simulink model "OMSv1_2x"  (Simulink 6.5)
settings: Solver=ode4  SolverMode=SingleTasking  StartTime=0.0  StopTime=5  FixedStep=0.001  MaxStep=0.001  RelTol=1e-3  AbsTol=1e-3
undefined symbols (not defined in the file): alexlaw, bs_onoff, bs_scale, bsfsacrit, bsfsvcrit, cnsgain, fs_onoff, fs_scale, fsdelaycalc, ltdrk, phasicgain, pmcgain, pmctau2, pmctau3, saccsw, spgain, tonicgain, tvrD, tvrN
libraries: simulink_extras x37
(part 4 of 5)

== system OMSv1_2x/OMS v1.2  07/21/05/IM CN-LMLN/Saccade Enable/Ret FB sample/event timer2 ==
  note: Resettable
      | Event Timer
  note: (Init input: 0)
  note: (FF init state: Q=0)
  note: (Init input: 0)
  note: In 2) Subsequent events DO NOT reset the counter; it only resets when it
      | reaches zero
  note: 2) A new event (leading or trailing edge) is detected. -- Only case 1)
  note: 1) The count reaches its limit (set in "timer value") -- Both case 1) and 2)
  note: In 1), A leading or trailing edge will reset the counter so that it
      | counts down from the end trailing edge) of that event.
  note: It has TWO modes: 1) Event resettable and 2) Event Non-resettable
  note: The real trick here is understanding how to reload the countdown.
      | It resets if either of two conditions is met:
  note: The "OR" gate allows either of these conditions to reset the circuit.  The delay before the
      | "S" input of the flip-flop prevents both "S" and "R" from being set simultaneously, because
      | this would put the flip-flop in an undefined state.
  note: Therefore, an event first RESETS and then SETS the flip-flop.
  note: This block is an RESETTABLE EVENT TIMER.  It outputs a spike of unit height xx milliseconds
      | (set by "timer value") after it detects an event ( i.e a TRAILING edge which represents the end of a
      |  saccadic pulse)
  RetFB EnCntrl : Inport
  _timer value (port) : Inport  Port=2
  1 msec : TransportDelay  DelayTime=.001
  Clock : Clock
      settings: Decimation=10
  Latch1 : simulink_extras/Flip Flops/S-R Flip-Flop  SystemSampleTime=-1  initial_condition=0
  Logical Operator : Logic  Operator=OR  Inputs=3
  Logical Operator1 : Logic
  Logical Operator2 : Logic
  Relational Operator : RelationalOperator  InputSameDT=on
  SampHold?1 : Subsystem
      mask Display: disp('S&H\n(S=L)\n(H=H)')
  Sum : Sum  Inputs=+-  SaturateOnIntegerOverflow=on  InputSameDT=on
  Terminator : Terminator
  event resettable? : Constant  Orientation=up
  leading edge detect : Subsystem
      mask Display: disp('Leading\nEdge Det')
  loop breaker : Memory  Orientation=left
  trailing edge detect : Subsystem
      mask Display: disp('Trailing\nEdge Det')
  outFF : Outport  InitialOutput=0
  wires:
  RetFB EnCntrl/1 -> trailing edge detect/1(in_1), leading edge detect/1(in_1)
  event resettable?/1 -> Logical Operator1/2, Logical Operator2/2
  leading edge detect/1(out_1) -> Logical Operator2/1
  Logical Operator2/1 -> Logical Operator/2
  trailing edge detect/1(out_1) -> 1 msec/1, Logical Operator1/1
  Logical Operator1/1 -> Logical Operator/1
  loop breaker/1 -> Logical Operator/3
  Latch1/1 -> SampHold?1/2(S/H?)
  Sum/1 -> Relational Operator/1
  Clock/1 -> SampHold?1/1(Input), Sum/1
  Relational Operator/1 -> outFF/1, loop breaker/1
  SampHold?1/1(output) -> Sum/2
  Logical Operator/1 -> Latch1/2
  1 msec/1 -> Latch1/1
  _timer value (port)/1 -> Relational Operator/2
  Latch1/2 -> Terminator/1

== system OMSv1_2x/OMS v1.2  07/21/05/IM CN-LMLN/Saccade Enable/Ret FB sample/event timer3 ==
  note: This block is an RESETTABLE EVENT TIMER.  It outputs a spike of unit height xx milliseconds
      | (set by "timer value") after it detects an event ( i.e a TRAILING edge which represents the end of a
      |  saccadic pulse)
  note: Therefore, an event first RESETS and then SETS the flip-flop.
  note: The "OR" gate allows either of these conditions to reset the circuit.  The delay before the
      | "S" input of the flip-flop prevents both "S" and "R" from being set simultaneously, because
      | this would put the flip-flop in an undefined state.
  note: The real trick here is understanding how to reload the countdown.
      | It resets if either of two conditions is met:
  note: It has TWO modes: 1) Event resettable and 2) Event Non-resettable
  note: In 1), A leading or trailing edge will reset the counter so that it
      | counts down from the end trailing edge) of that event.
  note: 1) The count reaches its limit (set in "timer value") -- Both case 1) and 2)
  note: 2) A new event (leading or trailing edge) is detected. -- Only case 1)
  note: In 2) Subsequent events DO NOT reset the counter; it only resets when it
      | reaches zero
  note: (Init input: 0)
  note: (FF init state: Q=0)
  note: (Init input: 0)
  note: Resettable
      | Event Timer
  RetFB EnCntrl : Inport
  _timer value (port) : Inport  Port=2
  1 msec : TransportDelay  DelayTime=.001
  Clock : Clock
      settings: Decimation=10
  Latch1 : simulink_extras/Flip Flops/S-R Flip-Flop  SystemSampleTime=-1  initial_condition=0
  Logical Operator : Logic  Operator=OR  Inputs=3
  Logical Operator1 : Logic
  Logical Operator2 : Logic
  Relational Operator : RelationalOperator  InputSameDT=on
  SampHold?1 : Subsystem
      mask Display: disp('S&H\n(S=L)\n(H=H)')
  Sum : Sum  Inputs=+-  SaturateOnIntegerOverflow=on  InputSameDT=on
  Terminator : Terminator
  event resettable? : Constant  Orientation=up
  leading edge detect : Subsystem
      mask Display: disp('Leading\nEdge Det')
  loop breaker : Memory  Orientation=left
  trailing edge detect : Subsystem
      mask Display: disp('Trailing\nEdge Det')
  outFF : Outport  InitialOutput=0
  wires:
  _timer value (port)/1 -> Relational Operator/2
  1 msec/1 -> Latch1/1
  Logical Operator/1 -> Latch1/2
  SampHold?1/1(output) -> Sum/2
  Clock/1 -> SampHold?1/1(Input), Sum/1
  Sum/1 -> Relational Operator/1
  Relational Operator/1 -> loop breaker/1, outFF/1
  Latch1/1 -> SampHold?1/2(S/H?)
  loop breaker/1 -> Logical Operator/3
  Logical Operator1/1 -> Logical Operator/1
  trailing edge detect/1(out_1) -> 1 msec/1, Logical Operator1/1
  Logical Operator2/1 -> Logical Operator/2
  leading edge detect/1(out_1) -> Logical Operator2/1
  event resettable?/1 -> Logical Operator1/2, Logical Operator2/2
  RetFB EnCntrl/1 -> trailing edge detect/1(in_1), leading edge detect/1(in_1)
  Latch1/2 -> Terminator/1

== system OMSv1_2x/OMS v1.2  07/21/05/IM CN-LMLN/Saccade Enable/Ret FB sample/leading edge detect2 ==
  note: It is also possible to remove the SIGNUM function
      | and the '==', and replace them with a simple
      | switch with a threshold of (say) 150 or so.
  note: leading edge detection
  in_1 : Inport
  Abs : Abs  SaturateOnIntegerOverflow=on
  Derivative : Derivative
  Relational Operator : RelationalOperator  Operator===  InputSameDT=on
  Sign : Signum
  Threshold 1 : Constant
  out_1 : Outport  InitialOutput=0
  wires:
  Abs/1 -> Derivative/1
  Derivative/1 -> Sign/1
  Sign/1 -> Relational Operator/1
  Threshold 1/1 -> Relational Operator/2
  Relational Operator/1 -> out_1/1
  in_1/1 -> Abs/1

== system OMSv1_2x/OMS v1.2  07/21/05/IM CN-LMLN/Saccade Enable/Ret FB sample/leading edge detect3 ==
  note: leading edge detection
  note: It is also possible to remove the SIGNUM function
      | and the '==', and replace them with a simple
      | switch with a threshold of (say) 150 or so.
  in_1 : Inport
  Abs : Abs  SaturateOnIntegerOverflow=on
  Derivative : Derivative
  Relational Operator : RelationalOperator  Operator===  InputSameDT=on
  Sign : Signum
  Threshold 1 : Constant
  out_1 : Outport  InitialOutput=0
  wires:
  in_1/1 -> Abs/1
  Relational Operator/1 -> out_1/1
  Threshold 1/1 -> Relational Operator/2
  Sign/1 -> Relational Operator/1
  Derivative/1 -> Sign/1
  Abs/1 -> Derivative/1

== system OMSv1_2x/OMS v1.2  07/21/05/IM CN-LMLN/Saccade Enable/Ret FB sample/leading edge detect4 ==
  note: It is also possible to remove the SIGNUM function
      | and the '==', and replace them with a simple
      | switch with a threshold of (say) 150 or so.
  note: leading edge detection
  in_1 : Inport
  Abs : Abs  SaturateOnIntegerOverflow=on
  Derivative : Derivative
  Relational Operator : RelationalOperator  Operator===  InputSameDT=on
  Sign : Signum
  Threshold 1 : Constant
  out_1 : Outport  InitialOutput=0
  wires:
  Abs/1 -> Derivative/1
  Derivative/1 -> Sign/1
  Sign/1 -> Relational Operator/1
  Threshold 1/1 -> Relational Operator/2
  Relational Operator/1 -> out_1/1
  in_1/1 -> Abs/1

== system OMSv1_2x/OMS v1.2  07/21/05/IM CN-LMLN/Saccade Enable/prolong/SampHold?2 ==
  note: When "S/H?" is LOW, then "Input" is switched directly to the
      | output ("sample").  When "S/H?" is HIGH, the current output is
      | maintained ("hold").
  Input : Inport
  S/H? : Inport  Port=2
  Memory : Memory  Orientation=left
  Sign : Signum
  Switch2 : Switch  Threshold=0.5  SaturateOnIntegerOverflow=on  InputSameDT=on
  output : Outport  InitialOutput=0
  wires:
  Memory/1 -> Switch2/1
  Switch2/1 -> output/1, Memory/1
  Input/1 -> Switch2/3
  Sign/1 -> Switch2/2
  S/H?/1 -> Sign/1

== system OMSv1_2x/OMS v1.2  07/21/05/IM CN-LMLN/Saccade Enable/prolong/leading edge detect ==
  note: leading edge detection
  in_1 : Inport
  Abs : Abs  SaturateOnIntegerOverflow=on
  Derivative : Derivative
  Relational Operator : RelationalOperator  Operator===  InputSameDT=on
  Sign : Signum
  Threshold 1 : Constant
  out_1 : Outport  InitialOutput=0
  wires:
  Abs/1 -> Derivative/1
  Derivative/1 -> Sign/1
  Sign/1 -> Relational Operator/1
  Threshold 1/1 -> Relational Operator/2
  Relational Operator/1 -> out_1/1
  in_1/1 -> Abs/1

== system OMSv1_2x/OMS v1.2  07/21/05/IM CN-LMLN/Saccade Enable/prolong/trailing edge detect ==
  note: trailing edge detection
  note: It is also possible to remove the SIGNUM function
      | and the '==', and replace them with a simple
      | switch with a threshold of (say) 150 or so.
  in_1 : Inport
  Abs : Abs  SaturateOnIntegerOverflow=on
  Derivative : Derivative
  Relational Operator : RelationalOperator  Operator===  InputSameDT=on
  Sign : Signum
  Threshold 1 : Constant  Value=-1
  out_1 : Outport  InitialOutput=0
  wires:
  in_1/1 -> Abs/1
  Relational Operator/1 -> out_1/1
  Threshold 1/1 -> Relational Operator/2
  Sign/1 -> Relational Operator/1
  Derivative/1 -> Sign/1
  Abs/1 -> Derivative/1

== system OMSv1_2x/OMS v1.2  07/21/05/IM CN-LMLN/Saccade Motor Commmand/TCHNG Override/event timer2 ==
  note: In 2) Subsequent events DO NOT reset the counter; it only resets when it
      | reaches zero
  note: 2) A new event (leading or trailing edge) is detected. -- Only case 1)
  note: 1) The count reaches its limit (set in "timer value") -- Both case 1) and 2)
  note: In 1), Any event (leading or trailing edge) will reset the counter so that it
      | counts down from the end trailing edge) of that event.
  note: It has TWO modes: 1) Event resettable and 2) Event Non-resettable
  note: The real trick here is understanding how to reload the countdown.
      | It resets if either of two conditions is met:
  note: The "OR" gate allows either of these conditions to reset the circuit.  The delay before the
      | "S" input of the flip-flop prevents both "S" and "R" from being set simultaneously, because
      | this would put the flip-flop in an undefined state.
  note: Therefore, an event first RESETS and then SETS the flip-flop.
  note: (Init input: 0)
  note: (FF init state: Q=0)
  note: (Init input: 0)
  note: This block is an RESETTABLE EVENT TIMER.  It outputs a spike of unit height xx milliseconds
      | (set by "timer value") after it detects an event ( i.e a TRAILING edge which represents the end of a
      |  saccadic pulse)
  note: Resettable
      | Event Timer
  _PG : Inport
  _timer value (port) : Inport  Port=2
  1 msec : TransportDelay  DelayTime=.001
  Clock : Clock
      settings: Decimation=10
  Latch1 : simulink_extras/Flip Flops/S-R Flip-Flop  SystemSampleTime=-1  initial_condition=0
  Logical Operator : Logic  Operator=OR  Inputs=3
  Logical Operator1 : Logic
  Logical Operator2 : Logic
  Relational Operator : RelationalOperator  InputSameDT=on
  SampHold?1 : Subsystem
      mask Display: disp('S&H\n(S=L)\n(H=H)')
  Sum : Sum  Inputs=+-  SaturateOnIntegerOverflow=on  InputSameDT=on
  Terminator : Terminator
  event resettable? : Constant  Orientation=up  Value=0
  leading edge detect : Subsystem
      mask Display: disp('Leading\nEdge Det')
  loop breaker : Memory  Orientation=left
  trailing edge detect : Subsystem
      mask Display: disp('Trailing\nEdge Det')
  out_1 : Outport  InitialOutput=0
  wires:
  event resettable?/1 -> Logical Operator2/2, Logical Operator1/2
  leading edge detect/1(out_1) -> Logical Operator2/1
  Logical Operator2/1 -> Logical Operator/2
  trailing edge detect/1(out_1) -> Logical Operator1/1, 1 msec/1
  Logical Operator1/1 -> Logical Operator/1
  loop breaker/1 -> Logical Operator/3
  _PG/1 -> leading edge detect/1(in_1), trailing edge detect/1(in_1)
  Latch1/1 -> SampHold?1/2(S/H?)
  Relational Operator/1 -> out_1/1, loop breaker/1
  Sum/1 -> Relational Operator/1
  Clock/1 -> Sum/1, SampHold?1/1(Input)
  SampHold?1/1(output) -> Sum/2
  Logical Operator/1 -> Latch1/2
  1 msec/1 -> Latch1/1
  _timer value (port)/1 -> Relational Operator/2
  Latch1/2 -> Terminator/1

== system OMSv1_2x/OMS v1.2  07/21/05/IM CN-LMLN/Saccade Motor Commmand/TCHNG Override/leading edge detect ==
  note: leading edge detection
  in_1 : Inport
  Abs : Abs  SaturateOnIntegerOverflow=on
  Derivative : Derivative
  Relational Operator : RelationalOperator  Operator===  InputSameDT=on
  Sign : Signum
  Threshold 1 : Constant
  out_1 : Outport  InitialOutput=0
  wires:
  in_1/1 -> Abs/1
  Relational Operator/1 -> out_1/1
  Threshold 1/1 -> Relational Operator/2
  Sign/1 -> Relational Operator/1
  Derivative/1 -> Sign/1
  Abs/1 -> Derivative/1

== system OMSv1_2x/OMS v1.2  07/21/05/IM CN-LMLN/Sampled Target Reconstruction/prolong/SampHold?2 ==
  note: When "S/H?" is LOW, then "Input" is switched directly to the
      | output ("sample").  When "S/H?" is HIGH, the current output is
      | maintained ("hold").
  Input : Inport
  S/H? : Inport  Port=2
  Memory : Memory  Orientation=left
  Sign : Signum
  Switch2 : Switch  Threshold=0.5  SaturateOnIntegerOverflow=on  InputSameDT=on
  output : Outport  InitialOutput=0
  wires:
  S/H?/1 -> Sign/1
  Sign/1 -> Switch2/2
  Input/1 -> Switch2/3
  Switch2/1 -> Memory/1, output/1
  Memory/1 -> Switch2/1

== system OMSv1_2x/OMS v1.2  07/21/05/IM CN-LMLN/Sampled Target Reconstruction/prolong/leading edge detect ==
  note: leading edge detection
  in_1 : Inport
  Abs : Abs  SaturateOnIntegerOverflow=on
  Derivative : Derivative
  Relational Operator : RelationalOperator  Operator===  InputSameDT=on
  Sign : Signum
  Threshold 1 : Constant
  out_1 : Outport  InitialOutput=0
  wires:
  in_1/1 -> Abs/1
  Relational Operator/1 -> out_1/1
  Threshold 1/1 -> Relational Operator/2
  Sign/1 -> Relational Operator/1
  Derivative/1 -> Sign/1
  Abs/1 -> Derivative/1

== system OMSv1_2x/OMS v1.2  07/21/05/IM CN-LMLN/Sampled Target Reconstruction/prolong/trailing edge detect ==
  note: It is also possible to remove the SIGNUM function
      | and the '==', and replace them with a simple
      | switch with a threshold of (say) 150 or so.
  note: trailing edge detection
  in_1 : Inport
  Abs : Abs  SaturateOnIntegerOverflow=on
  Derivative : Derivative
  Relational Operator : RelationalOperator  Operator===  InputSameDT=on
  Sign : Signum
  Threshold 1 : Constant  Value=-1
  out_1 : Outport  InitialOutput=0
  wires:
  Abs/1 -> Derivative/1
  Derivative/1 -> Sign/1
  Sign/1 -> Relational Operator/1
  Threshold 1/1 -> Relational Operator/2
  Relational Operator/1 -> out_1/1
  in_1/1 -> Abs/1

== system OMSv1_2x/OMS v1.2  07/21/05/IM CN-LMLN/Sampled Target Reconstruction/prolong1/SampHold?2 ==
  note: When "S/H?" is LOW, then "Input" is switched directly to the
      | output ("sample").  When "S/H?" is HIGH, the current output is
      | maintained ("hold").
  Input : Inport
  S/H? : Inport  Port=2
  Memory : Memory  Orientation=left
  Sign : Signum
  Switch2 : Switch  Threshold=0.5  SaturateOnIntegerOverflow=on  InputSameDT=on
  output : Outport  InitialOutput=0
  wires:
  Memory/1 -> Switch2/1
  Switch2/1 -> output/1, Memory/1
  Input/1 -> Switch2/3
  Sign/1 -> Switch2/2
  S/H?/1 -> Sign/1

== system OMSv1_2x/OMS v1.2  07/21/05/IM CN-LMLN/Sampled Target Reconstruction/prolong1/leading edge detect ==
  note: leading edge detection
  in_1 : Inport
  Abs : Abs  SaturateOnIntegerOverflow=on
  Derivative : Derivative
  Relational Operator : RelationalOperator  Operator===  InputSameDT=on
  Sign : Signum
  Threshold 1 : Constant
  out_1 : Outport  InitialOutput=0
  wires:
  Abs/1 -> Derivative/1
  Derivative/1 -> Sign/1
  Sign/1 -> Relational Operator/1
  Threshold 1/1 -> Relational Operator/2
  Relational Operator/1 -> out_1/1
  in_1/1 -> Abs/1

== system OMSv1_2x/OMS v1.2  07/21/05/IM CN-LMLN/Sampled Target Reconstruction/prolong1/trailing edge detect ==
  note: trailing edge detection
  note: It is also possible to remove the SIGNUM function
      | and the '==', and replace them with a simple
      | switch with a threshold of (say) 150 or so.
  in_1 : Inport
  Abs : Abs  SaturateOnIntegerOverflow=on
  Derivative : Derivative
  Relational Operator : RelationalOperator  Operator===  InputSameDT=on
  Sign : Signum
  Threshold 1 : Constant  Value=-1
  out_1 : Outport  InitialOutput=0
  wires:
  in_1/1 -> Abs/1
  Relational Operator/1 -> out_1/1
  Threshold 1/1 -> Relational Operator/2
  Sign/1 -> Relational Operator/1
  Derivative/1 -> Sign/1
  Abs/1 -> Derivative/1

== system OMSv1_2x/OMS v1.2  07/21/05/IM CN-LMLN/Sampled Target Reconstruction/prolong2/SampHold?2 ==
  note: When "S/H?" is LOW, then "Input" is switched directly to the
      | output ("sample").  When "S/H?" is HIGH, the current output is
      | maintained ("hold").
  Input : Inport
  S/H? : Inport  Port=2
  Memory : Memory  Orientation=left
  Sign : Signum
  Switch2 : Switch  Threshold=0.5  SaturateOnIntegerOverflow=on  InputSameDT=on
  output : Outport  InitialOutput=0
  wires:
  S/H?/1 -> Sign/1
  Sign/1 -> Switch2/2
  Input/1 -> Switch2/3
  Switch2/1 -> Memory/1, output/1
  Memory/1 -> Switch2/1

== system OMSv1_2x/OMS v1.2  07/21/05/IM CN-LMLN/Sampled Target Reconstruction/prolong2/leading edge detect ==
  note: leading edge detection
  in_1 : Inport
  Abs : Abs  SaturateOnIntegerOverflow=on
  Derivative : Derivative
  Relational Operator : RelationalOperator  Operator===  InputSameDT=on
  Sign : Signum
  Threshold 1 : Constant
  out_1 : Outport  InitialOutput=0
  wires:
  in_1/1 -> Abs/1
  Relational Operator/1 -> out_1/1
  Threshold 1/1 -> Relational Operator/2
  Sign/1 -> Relational Operator/1
  Derivative/1 -> Sign/1
  Abs/1 -> Derivative/1

== system OMSv1_2x/OMS v1.2  07/21/05/IM CN-LMLN/Sampled Target Reconstruction/prolong2/trailing edge detect ==
  note: It is also possible to remove the SIGNUM function
      | and the '==', and replace them with a simple
      | switch with a threshold of (say) 150 or so.
  note: trailing edge detection
  in_1 : Inport
  Abs : Abs  SaturateOnIntegerOverflow=on
  Derivative : Derivative
  Relational Operator : RelationalOperator  Operator===  InputSameDT=on
  Sign : Signum
  Threshold 1 : Constant  Value=-1
  out_1 : Outport  InitialOutput=0
  wires:
  Abs/1 -> Derivative/1
  Derivative/1 -> Sign/1
  Sign/1 -> Relational Operator/1
  Threshold 1/1 -> Relational Operator/2
  Relational Operator/1 -> out_1/1
  in_1/1 -> Abs/1

== system OMSv1_2x/OMS v1.2  07/21/05/PG w rNI1/PW funct/Input Switch/lead/trail edge det ==
  note: It is also possible to remove the SIGNUM function
      | and the '==', and replace them with a simple
      | switch with a threshold of (say) 150 or so.
  note: leading/trailing edge detection
  in_1 : Inport
  Abs : Abs  SaturateOnIntegerOverflow=on
  Derivative : Derivative
  Relational Operator : RelationalOperator  Operator===  InputSameDT=on
  Sign : Signum
  Threshold 1 : Constant
  out_1 : Outport  InitialOutput=0
  wires:
  Abs/1 -> Relational Operator/1
  Sign/1 -> Abs/1
  Derivative/1 -> Sign/1
  Threshold 1/1 -> Relational Operator/2
  Relational Operator/1 -> out_1/1
  in_1/1 -> Derivative/1

== system OMSv1_2x/OMS v1.2  07/21/05/PG w rNI1/RefLatch (Default = 50ms)/trailing edge/trailing edge det ==
  note: It is also possible to remove the SIGNUM function
      | and the '==', and replace them with a simple
      | switch with a threshold of (say) 150 or so.
  note: trailing edge detection
  in_1 : Inport
  Abs : Abs  SaturateOnIntegerOverflow=on
  Derivative : Derivative
  Relational Operator : RelationalOperator  Operator===  InputSameDT=on
  Sign : Signum
  Threshold 1 : Constant  Value=-1
  out_1 : Outport  InitialOutput=0
  wires:
  Abs/1 -> Derivative/1
  Derivative/1 -> Sign/1
  Sign/1 -> Relational Operator/1
  Threshold 1/1 -> Relational Operator/2
  Relational Operator/1 -> out_1/1
  in_1/1 -> Abs/1

== system OMSv1_2x/OMS v1.2  07/21/05/PG w rNI1/RefLatch (Default = 50ms)/trailing edge/trailing edge det1 ==
  note: trailing edge detection
  note: It is also possible to remove the SIGNUM function
      | and the '==', and replace them with a simple
      | switch with a threshold of (say) 150 or so.
  in_1 : Inport
  Abs : Abs  SaturateOnIntegerOverflow=on
  Derivative : Derivative
  Relational Operator : RelationalOperator  Operator===  InputSameDT=on
  Sign : Signum
  Threshold 1 : Constant  Value=-1
  out_1 : Outport  InitialOutput=0
  wires:
  in_1/1 -> Abs/1
  Relational Operator/1 -> out_1/1
  Threshold 1/1 -> Relational Operator/2
  Sign/1 -> Relational Operator/1
  Derivative/1 -> Sign/1
  Abs/1 -> Derivative/1

== system OMSv1_2x/OMS v1.2  07/21/05/IM CN-LMLN/BS/FS Logic/BS Enable1/BS Timing/event timer2 ==
  note: In 2) Subsequent events DO NOT reset the counter; it only resets when it
      | reaches zero
  note: 2) A new event (leading or trailing edge) is detected. -- Only case 1)
  note: 1) The count reaches its limit (set in "timer value") -- Both case 1) and 2)
  note: In 1), Any event (leading or trailing edge) will reset the counter so that it
      | counts down from the end trailing edge) of that event.
  note: It has TWO modes: 1) Event resettable and 2) Event Non-resettable
  note: The real trick here is understanding how to reload the countdown.
      | It resets if either of two conditions is met:
  note: The "OR" gate allows either of these conditions to reset the circuit.  The delay before the
      | "S" input of the flip-flop prevents both "S" and "R" from being set simultaneously, because
      | this would put the flip-flop in an undefined state.
  note: Therefore, an event first RESETS and then SETS the flip-flop.
  note: (Init input: 0)
  note: (FF init state: Q=0)
  note: (Init input: 0)
  note: This block is an RESETTABLE EVENT TIMER.  It outputs a spike of unit height xx milliseconds
      | (set by "timer value") after it detects an event ( i.e a TRAILING edge which represents the end of a
      |  saccadic pulse)
  note: Resettable
      | Event Timer
  _PG : Inport
  _timer value (port) : Inport  Port=2
  1 msec : TransportDelay  DelayTime=.001
  Clock : Clock
      settings: Decimation=10
  Latch1 : simulink_extras/Flip Flops/S-R Flip-Flop  SystemSampleTime=-1  initial_condition=0
  Logical Operator : Logic  Operator=OR  Inputs=3
  Logical Operator1 : Logic
  Logical Operator2 : Logic
  Relational Operator : RelationalOperator  InputSameDT=on
  SampHold?1 : Subsystem
      mask Display: disp('S&H\n(S=L)\n(H=H)')
  Sum : Sum  Inputs=+-  SaturateOnIntegerOverflow=on  InputSameDT=on
  Terminator : Terminator
  event resettable? : Constant  Orientation=up  Value=0
  leading edge detect : Subsystem
      mask Display: disp('Leading\nEdge Det')
  loop breaker : Memory  Orientation=left
  trailing edge detect : Subsystem
      mask Display: disp('Trailing\nEdge Det')
  out_1 : Outport  InitialOutput=0
  wires:
  event resettable?/1 -> Logical Operator2/2, Logical Operator1/2
  leading edge detect/1(out_1) -> Logical Operator2/1
  Logical Operator2/1 -> Logical Operator/2
  trailing edge detect/1(out_1) -> Logical Operator1/1, 1 msec/1
  Logical Operator1/1 -> Logical Operator/1
  loop breaker/1 -> Logical Operator/3
  _PG/1 -> leading edge detect/1(in_1), trailing edge detect/1(in_1)
  Latch1/1 -> SampHold?1/2(S/H?)
  Relational Operator/1 -> out_1/1, loop breaker/1
  Sum/1 -> Relational Operator/1
  Clock/1 -> Sum/1, SampHold?1/1(Input)
  SampHold?1/1(output) -> Sum/2
  Logical Operator/1 -> Latch1/2
  1 msec/1 -> Latch1/1
  _timer value (port)/1 -> Relational Operator/2
  Latch1/2 -> Terminator/1

== system OMSv1_2x/OMS v1.2  07/21/05/IM CN-LMLN/BS/FS Logic/BS Enable1/BS Timing/leading edge detect ==
  note: leading edge detection
  in_1 : Inport
  Abs : Abs  SaturateOnIntegerOverflow=on
  Derivative : Derivative
  Relational Operator : RelationalOperator  Operator===  InputSameDT=on
  Sign : Signum
  Threshold 1 : Constant
  out_1 : Outport  InitialOutput=0
  wires:
  in_1/1 -> Abs/1
  Relational Operator/1 -> out_1/1
  Threshold 1/1 -> Relational Operator/2
  Sign/1 -> Relational Operator/1
  Derivative/1 -> Sign/1
  Abs/1 -> Derivative/1

== system OMSv1_2x/OMS v1.2  07/21/05/IM CN-LMLN/BS/FS Logic/FS Enable/FS Timing/event timer2 ==
  note: Resettable
      | Event Timer
  note: This block is an RESETTABLE EVENT TIMER.  It outputs a spike of unit height xx milliseconds
      | (set by "timer value") after it detects an event ( i.e a TRAILING edge which represents the end of a
      |  saccadic pulse)
  note: (Init input: 0)
  note: (FF init state: Q=0)
  note: (Init input: 0)
  note: Therefore, an event first RESETS and then SETS the flip-flop.
  note: The "OR" gate allows either of these conditions to reset the circuit.  The delay before the
      | "S" input of the flip-flop prevents both "S" and "R" from being set simultaneously, because
      | this would put the flip-flop in an undefined state.
  note: The real trick here is understanding how to reload the countdown.
      | It resets if either of two conditions is met:
  note: It has TWO modes: 1) Event resettable and 2) Event Non-resettable
  note: In 1), Any event (leading or trailing edge) will reset the counter so that it
      | counts down from the end trailing edge) of that event.
  note: 1) The count reaches its limit (set in "timer value") -- Both case 1) and 2)
  note: 2) A new event (leading or trailing edge) is detected. -- Only case 1)
  note: In 2) Subsequent events DO NOT reset the counter; it only resets when it
      | reaches zero
  _PG : Inport
  _timer value (port) : Inport  Port=2
  1 msec : TransportDelay  DelayTime=.001
  Clock : Clock
      settings: Decimation=10
  Latch1 : simulink_extras/Flip Flops/S-R Flip-Flop  SystemSampleTime=-1  initial_condition=0
  Logical Operator : Logic  Operator=OR  Inputs=3
  Logical Operator1 : Logic
  Logical Operator2 : Logic
  Relational Operator : RelationalOperator  InputSameDT=on
  SampHold?1 : Subsystem
      mask Display: disp('S&H\n(S=L)\n(H=H)')
  Sum : Sum  Inputs=+-  SaturateOnIntegerOverflow=on  InputSameDT=on
  Terminator : Terminator
  event resettable? : Constant  Orientation=up  Value=0
  leading edge detect : Subsystem
      mask Display: disp('Leading\nEdge Det')
  loop breaker : Memory  Orientation=left
  trailing edge detect : Subsystem
      mask Display: disp('Trailing\nEdge Det')
  out_1 : Outport  InitialOutput=0
  wires:
  _timer value (port)/1 -> Relational Operator/2
  1 msec/1 -> Latch1/1
  Logical Operator/1 -> Latch1/2
  SampHold?1/1(output) -> Sum/2
  Clock/1 -> SampHold?1/1(Input), Sum/1
  Sum/1 -> Relational Operator/1
  Relational Operator/1 -> loop breaker/1, out_1/1
  Latch1/1 -> SampHold?1/2(S/H?)
  _PG/1 -> trailing edge detect/1(in_1), leading edge detect/1(in_1)
  loop breaker/1 -> Logical Operator/3
  Logical Operator1/1 -> Logical Operator/1
  trailing edge detect/1(out_1) -> 1 msec/1, Logical Operator1/1
  Logical Operator2/1 -> Logical Operator/2
  leading edge detect/1(out_1) -> Logical Operator2/1
  event resettable?/1 -> Logical Operator1/2, Logical Operator2/2
  Latch1/2 -> Terminator/1

== system OMSv1_2x/OMS v1.2  07/21/05/IM CN-LMLN/BS/FS Logic/FS Enable/FS Timing/leading edge detect ==
  note: leading edge detection
  in_1 : Inport
  Abs : Abs  SaturateOnIntegerOverflow=on
  Derivative : Derivative
  Relational Operator : RelationalOperator  Operator===  InputSameDT=on
  Sign : Signum
  Threshold 1 : Constant
  out_1 : Outport  InitialOutput=0
  wires:
  Abs/1 -> Derivative/1
  Derivative/1 -> Sign/1
  Sign/1 -> Relational Operator/1
  Threshold 1/1 -> Relational Operator/2
  Relational Operator/1 -> out_1/1
  in_1/1 -> Abs/1

== system OMSv1_2x/OMS v1.2  07/21/05/IM CN-LMLN/BS/FS Logic/TCHNG Override/event timer2/SampHold?1 ==
  note: When "S/H?" is LOW, then "Input" is switched directly to the
      | output ("sample").  When "S/H?" is HIGH, the current output is
      | maintained ("hold").
  Input : Inport
  S/H? : Inport  Port=2
  Memory : Memory  Orientation=left
  Sign : Signum
  Switch2 : Switch  Threshold=0.5  SaturateOnIntegerOverflow=on  InputSameDT=on
  output : Outport  InitialOutput=0
  wires:
  Switch2/1 -> Memory/1, output/1
  Sign/1 -> Switch2/2
  S/H?/1 -> Sign/1
  Memory/1 -> Switch2/1
  Input/1 -> Switch2/3

== system OMSv1_2x/OMS v1.2  07/21/05/IM CN-LMLN/BS/FS Logic/TCHNG Override/event timer2/leading edge detect ==
  note: It is also possible to remove the SIGNUM function
      | and the '==', and replace them with a simple
      | switch with a threshold of (say) 150 or so.
  note: leading edge detection
  in_1 : Inport
  Abs : Abs  SaturateOnIntegerOverflow=on
  Derivative : Derivative
  Relational Operator : RelationalOperator  Operator===  InputSameDT=on
  Sign : Signum
  Threshold 1 : Constant
  out_1 : Outport  InitialOutput=0
  wires:
  Abs/1 -> Derivative/1
  Derivative/1 -> Sign/1
  Sign/1 -> Relational Operator/1
  Threshold 1/1 -> Relational Operator/2
  Relational Operator/1 -> out_1/1
  in_1/1 -> Abs/1

== system OMSv1_2x/OMS v1.2  07/21/05/IM CN-LMLN/BS/FS Logic/TCHNG Override/event timer2/trailing edge detect ==
  note: trailing edge detection
  note: It is also possible to remove the SIGNUM function
      | and the '==', and replace them with a simple
      | switch with a threshold of (say) 150 or so.
  in_1 : Inport
  Abs : Abs  SaturateOnIntegerOverflow=on
  Derivative : Derivative
  Relational Operator : RelationalOperator  Operator===  InputSameDT=on
  Sign : Signum
  Threshold 1 : Constant  Value=-1
  out_1 : Outport  InitialOutput=0
  wires:
  in_1/1 -> Abs/1
  Relational Operator/1 -> out_1/1
  Threshold 1/1 -> Relational Operator/2
  Sign/1 -> Relational Operator/1
  Derivative/1 -> Sign/1
  Abs/1 -> Derivative/1

== system OMSv1_2x/OMS v1.2  07/21/05/IM CN-LMLN/Saccade Enable/Enable Control/2 ms/SampHold?2 ==
  note: When "S/H?" is LOW, then "Input" is switched directly to the
      | output ("sample").  When "S/H?" is HIGH, the current output is
      | maintained ("hold").
  Input : Inport
  S/H? : Inport  Port=2
  Memory : Memory  Orientation=left
  Sign : Signum
  Switch2 : Switch  Threshold=0.5  SaturateOnIntegerOverflow=on  InputSameDT=on
  output : Outport  InitialOutput=0
  wires:
  Memory/1 -> Switch2/1
  Switch2/1 -> output/1, Memory/1
  Input/1 -> Switch2/3
  Sign/1 -> Switch2/2
  S/H?/1 -> Sign/1

== system OMSv1_2x/OMS v1.2  07/21/05/IM CN-LMLN/Saccade Enable/Enable Control/2 ms/leading edge detect ==
  note: leading edge detection
  in_1 : Inport
  Abs : Abs  SaturateOnIntegerOverflow=on
  Derivative : Derivative
  Relational Operator : RelationalOperator  Operator===  InputSameDT=on
  Sign : Signum
  Threshold 1 : Constant
  out_1 : Outport  InitialOutput=0
  wires:
  Abs/1 -> Derivative/1
  Derivative/1 -> Sign/1
  Sign/1 -> Relational Operator/1
  Threshold 1/1 -> Relational Operator/2
  Relational Operator/1 -> out_1/1
  in_1/1 -> Abs/1

== system OMSv1_2x/OMS v1.2  07/21/05/IM CN-LMLN/Saccade Enable/Enable Control/2 ms/trailing edge detect ==
  note: trailing edge detection
  note: It is also possible to remove the SIGNUM function
      | and the '==', and replace them with a simple
      | switch with a threshold of (say) 150 or so.
  in_1 : Inport
  Abs : Abs  SaturateOnIntegerOverflow=on
  Derivative : Derivative
  Relational Operator : RelationalOperator  Operator===  InputSameDT=on
  Sign : Signum
  Threshold 1 : Constant  Value=-1
  out_1 : Outport  InitialOutput=0
  wires:
  in_1/1 -> Abs/1
  Relational Operator/1 -> out_1/1
  Threshold 1/1 -> Relational Operator/2
  Sign/1 -> Relational Operator/1
  Derivative/1 -> Sign/1
  Abs/1 -> Derivative/1

== system OMSv1_2x/OMS v1.2  07/21/05/IM CN-LMLN/Saccade Enable/Enable Control/50 ms/SampHold?2 ==
  note: When "S/H?" is LOW, then "Input" is switched directly to the
      | output ("sample").  When "S/H?" is HIGH, the current output is
      | maintained ("hold").
  Input : Inport
  S/H? : Inport  Port=2
  Memory : Memory  Orientation=left
  Sign : Signum
  Switch2 : Switch  Threshold=0.5  SaturateOnIntegerOverflow=on  InputSameDT=on
  output : Outport  InitialOutput=0
  wires:
  S/H?/1 -> Sign/1
  Sign/1 -> Switch2/2
  Input/1 -> Switch2/3
  Switch2/1 -> Memory/1, output/1
  Memory/1 -> Switch2/1

== system OMSv1_2x/OMS v1.2  07/21/05/IM CN-LMLN/Saccade Enable/Enable Control/50 ms/leading edge detect ==
  note: leading edge detection
  in_1 : Inport
  Abs : Abs  SaturateOnIntegerOverflow=on
  Derivative : Derivative
  Relational Operator : RelationalOperator  Operator===  InputSameDT=on
  Sign : Signum
  Threshold 1 : Constant
  out_1 : Outport  InitialOutput=0
  wires:
  in_1/1 -> Abs/1
  Relational Operator/1 -> out_1/1
  Threshold 1/1 -> Relational Operator/2
  Sign/1 -> Relational Operator/1
  Derivative/1 -> Sign/1
  Abs/1 -> Derivative/1

== system OMSv1_2x/OMS v1.2  07/21/05/IM CN-LMLN/Saccade Enable/Enable Control/50 ms/trailing edge detect ==
  note: It is also possible to remove the SIGNUM function
      | and the '==', and replace them with a simple
      | switch with a threshold of (say) 150 or so.
  note: trailing edge detection
  in_1 : Inport
  Abs : Abs  SaturateOnIntegerOverflow=on
  Derivative : Derivative
  Relational Operator : RelationalOperator  Operator===  InputSameDT=on
  Sign : Signum
  Threshold 1 : Constant  Value=-1
  out_1 : Outport  InitialOutput=0
  wires:
  Abs/1 -> Derivative/1
  Derivative/1 -> Sign/1
  Sign/1 -> Relational Operator/1
  Threshold 1/1 -> Relational Operator/2
  Relational Operator/1 -> out_1/1
  in_1/1 -> Abs/1

== system OMSv1_2x/OMS v1.2  07/21/05/IM CN-LMLN/Saccade Enable/Enable Control/ECPY Timing/leading edge detect ==
  note: It is also possible to remove the SIGNUM function
      | and the '==', and replace them with a simple
      | switch with a threshold of (say) 150 or so.
  note: leading edge detection
  in_1 : Inport
  Abs : Abs  SaturateOnIntegerOverflow=on
  Derivative : Derivative
  Relational Operator : RelationalOperator  Operator===  InputSameDT=on
  Sign : Signum
  Threshold 1 : Constant
  out_1 : Outport  InitialOutput=0
  wires:
  Abs/1 -> Derivative/1
  Derivative/1 -> Sign/1
  Sign/1 -> Relational Operator/1
  Threshold 1/1 -> Relational Operator/2
  Relational Operator/1 -> out_1/1
  in_1/1 -> Abs/1

== system OMSv1_2x/OMS v1.2  07/21/05/IM CN-LMLN/Saccade Enable/Enable Control/ECPY Timing/leading edge detect1 ==
  note: leading edge detection
  note: It is also possible to remove the SIGNUM function
      | and the '==', and replace them with a simple
      | switch with a threshold of (say) 150 or so.
  in_1 : Inport
  Abs : Abs  SaturateOnIntegerOverflow=on
  Derivative : Derivative
  Relational Operator : RelationalOperator  Operator===  InputSameDT=on
  Sign : Signum
  Threshold 1 : Constant
  out_1 : Outport  InitialOutput=0
  wires:
  in_1/1 -> Abs/1
  Relational Operator/1 -> out_1/1
  Threshold 1/1 -> Relational Operator/2
  Sign/1 -> Relational Operator/1
  Derivative/1 -> Sign/1
  Abs/1 -> Derivative/1

== system OMSv1_2x/OMS v1.2  07/21/05/IM CN-LMLN/Saccade Enable/Enable Control/ECPY Timing/trailing edge detect ==
  note: trailing edge detection
  note: It is also possible to remove the SIGNUM function
      | and the '==', and replace them with a simple
      | switch with a threshold of (say) 150 or so.
  in_1 : Inport
  Abs : Abs  SaturateOnIntegerOverflow=on
  Derivative : Derivative
  Relational Operator : RelationalOperator  Operator===  InputSameDT=on
  Sign : Signum
  Threshold 1 : Constant  Value=-1
  out_1 : Outport  InitialOutput=0
  wires:
  in_1/1 -> Abs/1
  Relational Operator/1 -> out_1/1
  Threshold 1/1 -> Relational Operator/2
  Sign/1 -> Relational Operator/1
  Derivative/1 -> Sign/1
  Abs/1 -> Derivative/1

== system OMSv1_2x/OMS v1.2  07/21/05/IM CN-LMLN/Saccade Enable/Enable Control/event timer1/SampHold?1 ==
  note: When "S/H?" is LOW, then "Input" is switched directly to the
      | output ("sample").  When "S/H?" is HIGH, the current output is
      | maintained ("hold").
  Input : Inport
  S/H? : Inport  Port=2
  Memory : Memory  Orientation=left
  Sign : Signum
  Switch2 : Switch  Threshold=0.5  SaturateOnIntegerOverflow=on  InputSameDT=on
  output : Outport  InitialOutput=0
  wires:
  Input/1 -> Switch2/3
  Memory/1 -> Switch2/1
  S/H?/1 -> Sign/1
  Sign/1 -> Switch2/2
  Switch2/1 -> output/1, Memory/1

== system OMSv1_2x/OMS v1.2  07/21/05/IM CN-LMLN/Saccade Enable/Enable Control/event timer1/leading edge detect ==
  note: leading edge detection
  note: It is also possible to remove the SIGNUM function
      | and the '==', and replace them with a simple
      | switch with a threshold of (say) 150 or so.
  in_1 : Inport
  Abs : Abs  SaturateOnIntegerOverflow=on
  Derivative : Derivative
  Relational Operator : RelationalOperator  Operator===  InputSameDT=on
  Sign : Signum
  Threshold 1 : Constant
  out_1 : Outport  InitialOutput=0
  wires:
  in_1/1 -> Abs/1
  Relational Operator/1 -> out_1/1
  Threshold 1/1 -> Relational Operator/2
  Sign/1 -> Relational Operator/1
  Derivative/1 -> Sign/1
  Abs/1 -> Derivative/1

== system OMSv1_2x/OMS v1.2  07/21/05/IM CN-LMLN/Saccade Enable/Enable Control/event timer1/trailing edge detect ==
  note: It is also possible to remove the SIGNUM function
      | and the '==', and replace them with a simple
      | switch with a threshold of (say) 150 or so.
  note: trailing edge detection
  in_1 : Inport
  Abs : Abs  SaturateOnIntegerOverflow=on
  Derivative : Derivative
  Relational Operator : RelationalOperator  Operator===  InputSameDT=on
  Sign : Signum
  Threshold 1 : Constant  Value=-1
  out_1 : Outport  InitialOutput=0
  wires:
  Abs/1 -> Derivative/1
  Derivative/1 -> Sign/1
  Sign/1 -> Relational Operator/1
  Threshold 1/1 -> Relational Operator/2
  Relational Operator/1 -> out_1/1
  in_1/1 -> Abs/1

== system OMSv1_2x/OMS v1.2  07/21/05/IM CN-LMLN/Saccade Enable/LN FPh Gen/event timer1/SampHold?1 ==
  note: When "S/H?" is LOW, then "Input" is switched directly to the
      | output ("sample").  When "S/H?" is HIGH, the current output is
      | maintained ("hold").
  Input : Inport
  S/H? : Inport  Port=2
  Memory : Memory  Orientation=left
  Sign : Signum
  Switch2 : Switch  Threshold=0.5  SaturateOnIntegerOverflow=on  InputSameDT=on
  output : Outport  InitialOutput=0
  wires:
  Input/1 -> Switch2/3
  Memory/1 -> Switch2/1
  S/H?/1 -> Sign/1
  Sign/1 -> Switch2/2
  Switch2/1 -> output/1, Memory/1

== system OMSv1_2x/OMS v1.2  07/21/05/IM CN-LMLN/Saccade Enable/LN FPh Gen/event timer1/leading edge detect ==
  note: leading edge detection
  note: It is also possible to remove the SIGNUM function
      | and the '==', and replace them with a simple
      | switch with a threshold of (say) 150 or so.
  in_1 : Inport
  Abs : Abs  SaturateOnIntegerOverflow=on
  Derivative : Derivative
  Relational Operator : RelationalOperator  Operator===  InputSameDT=on
  Sign : Signum
  Threshold 1 : Constant
  out_1 : Outport  InitialOutput=0
  wires:
  in_1/1 -> Abs/1
  Relational Operator/1 -> out_1/1
  Threshold 1/1 -> Relational Operator/2
  Sign/1 -> Relational Operator/1
  Derivative/1 -> Sign/1
  Abs/1 -> Derivative/1

== system OMSv1_2x/OMS v1.2  07/21/05/IM CN-LMLN/Saccade Enable/LN FPh Gen/event timer1/trailing edge detect ==
  note: It is also possible to remove the SIGNUM function
      | and the '==', and replace them with a simple
      | switch with a threshold of (say) 150 or so.
  note: trailing edge detection
  in_1 : Inport
  Abs : Abs  SaturateOnIntegerOverflow=on
  Derivative : Derivative
  Relational Operator : RelationalOperator  Operator===  InputSameDT=on
  Sign : Signum
  Threshold 1 : Constant  Value=-1
  out_1 : Outport  InitialOutput=0
  wires:
  Abs/1 -> Derivative/1
  Derivative/1 -> Sign/1
  Sign/1 -> Relational Operator/1
  Threshold 1/1 -> Relational Operator/2
  Relational Operator/1 -> out_1/1
  in_1/1 -> Abs/1

== system OMSv1_2x/OMS v1.2  07/21/05/IM CN-LMLN/Saccade Enable/Ret FB sample/event timer2/SampHold?1 ==
  note: When "S/H?" is LOW, then "Input" is switched directly to the
      | output ("sample").  When "S/H?" is HIGH, the current output is
      | maintained ("hold").
  Input : Inport
  S/H? : Inport  Port=2
  Memory : Memory  Orientation=left
  Sign : Signum
  Switch2 : Switch  Threshold=0.5  SaturateOnIntegerOverflow=on  InputSameDT=on
  output : Outport  InitialOutput=0
  wires:
  Switch2/1 -> Memory/1, output/1
  Sign/1 -> Switch2/2
  S/H?/1 -> Sign/1
  Memory/1 -> Switch2/1
  Input/1 -> Switch2/3

== system OMSv1_2x/OMS v1.2  07/21/05/IM CN-LMLN/Saccade Enable/Ret FB sample/event timer2/leading edge detect ==
  note: It is also possible to remove the SIGNUM function
      | and the '==', and replace them with a simple
      | switch with a threshold of (say) 150 or so.
  note: leading edge detection
  in_1 : Inport
  Abs : Abs  SaturateOnIntegerOverflow=on
  Derivative : Derivative
  Relational Operator : RelationalOperator  Operator===  InputSameDT=on
  Sign : Signum
  Threshold 1 : Constant
  out_1 : Outport  InitialOutput=0
  wires:
  Abs/1 -> Derivative/1
  Derivative/1 -> Sign/1
  Sign/1 -> Relational Operator/1
  Threshold 1/1 -> Relational Operator/2
  Relational Operator/1 -> out_1/1
  in_1/1 -> Abs/1

== system OMSv1_2x/OMS v1.2  07/21/05/IM CN-LMLN/Saccade Enable/Ret FB sample/event timer2/trailing edge detect ==
  note: trailing edge detection
  note: It is also possible to remove the SIGNUM function
      | and the '==', and replace them with a simple
      | switch with a threshold of (say) 150 or so.
  in_1 : Inport
  Abs : Abs  SaturateOnIntegerOverflow=on
  Derivative : Derivative
  Relational Operator : RelationalOperator  Operator===  InputSameDT=on
  Sign : Signum
  Threshold 1 : Constant  Value=-1
  out_1 : Outport  InitialOutput=0
  wires:
  in_1/1 -> Abs/1
  Relational Operator/1 -> out_1/1
  Threshold 1/1 -> Relational Operator/2
  Sign/1 -> Relational Operator/1
  Derivative/1 -> Sign/1
  Abs/1 -> Derivative/1

== system OMSv1_2x/OMS v1.2  07/21/05/IM CN-LMLN/Saccade Enable/Ret FB sample/event timer3/SampHold?1 ==
  note: When "S/H?" is LOW, then "Input" is switched directly to the
      | output ("sample").  When "S/H?" is HIGH, the current output is
      | maintained ("hold").
  Input : Inport
  S/H? : Inport  Port=2
  Memory : Memory  Orientation=left
  Sign : Signum
  Switch2 : Switch  Threshold=0.5  SaturateOnIntegerOverflow=on  InputSameDT=on
  output : Outport  InitialOutput=0
  wires:
  Input/1 -> Switch2/3
  Memory/1 -> Switch2/1
  S/H?/1 -> Sign/1
  Sign/1 -> Switch2/2
  Switch2/1 -> output/1, Memory/1

== system OMSv1_2x/OMS v1.2  07/21/05/IM CN-LMLN/Saccade Enable/Ret FB sample/event timer3/leading edge detect ==
  note: leading edge detection
  note: It is also possible to remove the SIGNUM function
      | and the '==', and replace them with a simple
      | switch with a threshold of (say) 150 or so.
  in_1 : Inport
  Abs : Abs  SaturateOnIntegerOverflow=on
  Derivative : Derivative
  Relational Operator : RelationalOperator  Operator===  InputSameDT=on
  Sign : Signum
  Threshold 1 : Constant
  out_1 : Outport  InitialOutput=0
  wires:
  in_1/1 -> Abs/1
  Relational Operator/1 -> out_1/1
  Threshold 1/1 -> Relational Operator/2
  Sign/1 -> Relational Operator/1
  Derivative/1 -> Sign/1
  Abs/1 -> Derivative/1

== system OMSv1_2x/OMS v1.2  07/21/05/IM CN-LMLN/Saccade Enable/Ret FB sample/event timer3/trailing edge detect ==
  note: It is also possible to remove the SIGNUM function
      | and the '==', and replace them with a simple
      | switch with a threshold of (say) 150 or so.
  note: trailing edge detection
  in_1 : Inport
  Abs : Abs  SaturateOnIntegerOverflow=on
  Derivative : Derivative
  Relational Operator : RelationalOperator  Operator===  InputSameDT=on
  Sign : Signum
  Threshold 1 : Constant  Value=-1
  out_1 : Outport  InitialOutput=0
  wires:
  Abs/1 -> Derivative/1
  Derivative/1 -> Sign/1
  Sign/1 -> Relational Operator/1
  Threshold 1/1 -> Relational Operator/2
  Relational Operator/1 -> out_1/1
  in_1/1 -> Abs/1

== system OMSv1_2x/OMS v1.2  07/21/05/IM CN-LMLN/Saccade Motor Commmand/TCHNG Override/event timer2/SampHold?1 ==
  note: When "S/H?" is LOW, then "Input" is switched directly to the
      | output ("sample").  When "S/H?" is HIGH, the current output is
      | maintained ("hold").
  Input : Inport
  S/H? : Inport  Port=2
  Memory : Memory  Orientation=left
  Sign : Signum
  Switch2 : Switch  Threshold=0.5  SaturateOnIntegerOverflow=on  InputSameDT=on
  output : Outport  InitialOutput=0
  wires:
  Switch2/1 -> Memory/1, output/1
  Sign/1 -> Switch2/2
  S/H?/1 -> Sign/1
  Memory/1 -> Switch2/1
  Input/1 -> Switch2/3

== system OMSv1_2x/OMS v1.2  07/21/05/IM CN-LMLN/Saccade Motor Commmand/TCHNG Override/event timer2/leading edge detect ==
  note: It is also possible to remove the SIGNUM function
      | and the '==', and replace them with a simple
      | switch with a threshold of (say) 150 or so.
  note: leading edge detection
  in_1 : Inport
  Abs : Abs  SaturateOnIntegerOverflow=on
  Derivative : Derivative
  Relational Operator : RelationalOperator  Operator===  InputSameDT=on
  Sign : Signum
  Threshold 1 : Constant
  out_1 : Outport  InitialOutput=0
  wires:
  Abs/1 -> Derivative/1
  Derivative/1 -> Sign/1
  Sign/1 -> Relational Operator/1
  Threshold 1/1 -> Relational Operator/2
  Relational Operator/1 -> out_1/1
  in_1/1 -> Abs/1

== system OMSv1_2x/OMS v1.2  07/21/05/IM CN-LMLN/Saccade Motor Commmand/TCHNG Override/event timer2/trailing edge detect ==
  note: trailing edge detection
  note: It is also possible to remove the SIGNUM function
      | and the '==', and replace them with a simple
      | switch with a threshold of (say) 150 or so.
  in_1 : Inport
  Abs : Abs  SaturateOnIntegerOverflow=on
  Derivative : Derivative
  Relational Operator : RelationalOperator  Operator===  InputSameDT=on
  Sign : Signum
  Threshold 1 : Constant  Value=-1
  out_1 : Outport  InitialOutput=0
  wires:
  in_1/1 -> Abs/1
  Relational Operator/1 -> out_1/1
  Threshold 1/1 -> Relational Operator/2
  Sign/1 -> Relational Operator/1
  Derivative/1 -> Sign/1
  Abs/1 -> Derivative/1

== system OMSv1_2x/OMS v1.2  07/21/05/IM CN-LMLN/BS/FS Logic/BS Enable1/BS Timing/event timer2/SampHold?1 ==
  note: When "S/H?" is LOW, then "Input" is switched directly to the
      | output ("sample").  When "S/H?" is HIGH, the current output is
      | maintained ("hold").
  Input : Inport
  S/H? : Inport  Port=2
  Memory : Memory  Orientation=left
  Sign : Signum
  Switch2 : Switch  Threshold=0.5  SaturateOnIntegerOverflow=on  InputSameDT=on
  output : Outport  InitialOutput=0
  wires:
  Switch2/1 -> Memory/1, output/1
  Sign/1 -> Switch2/2
  S/H?/1 -> Sign/1
  Memory/1 -> Switch2/1
  Input/1 -> Switch2/3

== system OMSv1_2x/OMS v1.2  07/21/05/IM CN-LMLN/BS/FS Logic/BS Enable1/BS Timing/event timer2/leading edge detect ==
  note: It is also possible to remove the SIGNUM function
      | and the '==', and replace them with a simple
      | switch with a threshold of (say) 150 or so.
  note: leading edge detection
  in_1 : Inport
  Abs : Abs  SaturateOnIntegerOverflow=on
  Derivative : Derivative
  Relational Operator : RelationalOperator  Operator===  InputSameDT=on
  Sign : Signum
  Threshold 1 : Constant
  out_1 : Outport  InitialOutput=0
  wires:
  Abs/1 -> Derivative/1
  Derivative/1 -> Sign/1
  Sign/1 -> Relational Operator/1
  Threshold 1/1 -> Relational Operator/2
  Relational Operator/1 -> out_1/1
  in_1/1 -> Abs/1

== system OMSv1_2x/OMS v1.2  07/21/05/IM CN-LMLN/BS/FS Logic/BS Enable1/BS Timing/event timer2/trailing edge detect ==
  note: trailing edge detection
  note: It is also possible to remove the SIGNUM function
      | and the '==', and replace them with a simple
      | switch with a threshold of (say) 150 or so.
  in_1 : Inport
  Abs : Abs  SaturateOnIntegerOverflow=on
  Derivative : Derivative
  Relational Operator : RelationalOperator  Operator===  InputSameDT=on
  Sign : Signum
  Threshold 1 : Constant  Value=-1
  out_1 : Outport  InitialOutput=0
  wires:
  in_1/1 -> Abs/1
  Relational Operator/1 -> out_1/1
  Threshold 1/1 -> Relational Operator/2
  Sign/1 -> Relational Operator/1
  Derivative/1 -> Sign/1
  Abs/1 -> Derivative/1

== system OMSv1_2x/OMS v1.2  07/21/05/IM CN-LMLN/BS/FS Logic/FS Enable/FS Timing/event timer2/SampHold?1 ==
  note: When "S/H?" is LOW, then "Input" is switched directly to the
      | output ("sample").  When "S/H?" is HIGH, the current output is
      | maintained ("hold").
  Input : Inport
  S/H? : Inport  Port=2
  Memory : Memory  Orientation=left
  Sign : Signum
  Switch2 : Switch  Threshold=0.5  SaturateOnIntegerOverflow=on  InputSameDT=on
  output : Outport  InitialOutput=0
  wires:
  Input/1 -> Switch2/3
  Memory/1 -> Switch2/1
  S/H?/1 -> Sign/1
  Sign/1 -> Switch2/2
  Switch2/1 -> output/1, Memory/1

== system OMSv1_2x/OMS v1.2  07/21/05/IM CN-LMLN/BS/FS Logic/FS Enable/FS Timing/event timer2/leading edge detect ==
  note: leading edge detection
  note: It is also possible to remove the SIGNUM function
      | and the '==', and replace them with a simple
      | switch with a threshold of (say) 150 or so.
  in_1 : Inport
  Abs : Abs  SaturateOnIntegerOverflow=on
  Derivative : Derivative
  Relational Operator : RelationalOperator  Operator===  InputSameDT=on
  Sign : Signum
  Threshold 1 : Constant
  out_1 : Outport  InitialOutput=0
  wires:
  in_1/1 -> Abs/1
  Relational Operator/1 -> out_1/1
  Threshold 1/1 -> Relational Operator/2
  Sign/1 -> Relational Operator/1
  Derivative/1 -> Sign/1
  Abs/1 -> Derivative/1
